simulink model "example_C_simulation_of_nominal_case"  (R2017b)
settings: Solver=VariableStepAuto  StartTime=0.0  StopTime=0.5  MaxStep=1e-3  RelTol=1e-3
undefined symbols (not defined in the file): DiscIntNeverNeededParam
settings Model: Creator=user  LastModifiedBy=user

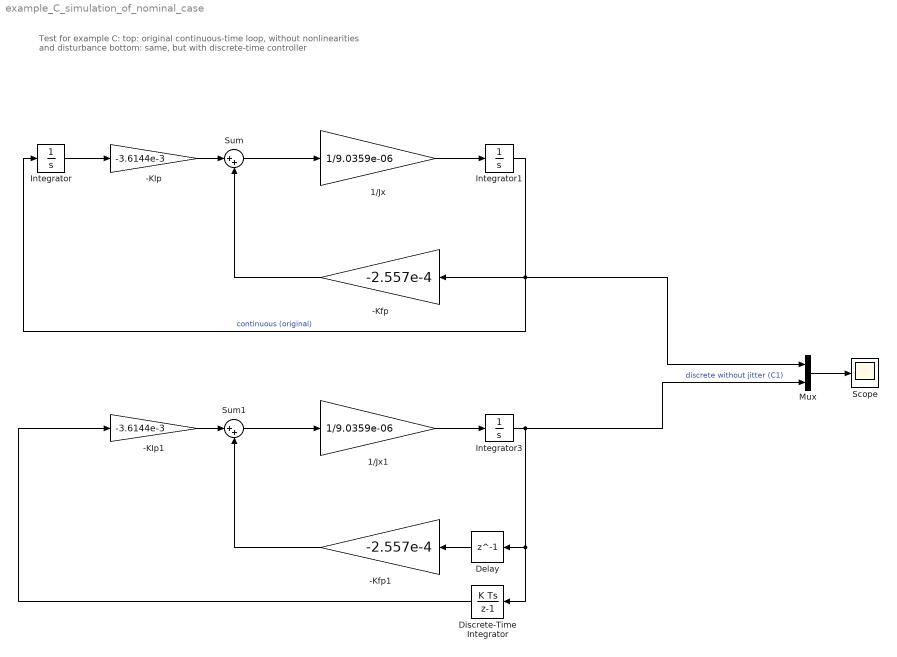
== system example_C_simulation_of_nominal_case ==
  note: Test for example C:
      | top: original continuous-time loop, without nonlinearities and disturbance
      | bottom: same, but with discrete-time controller
  -KIp : Gain  Gain=-3.6144e-3
  -KIp1 : Gain  Gain=-3.6144e-3
  -Kfp : Gain  Gain=-2.557e-4
  -Kfp1 : Gain  Gain=-2.557e-4
  1/Jx : Gain  Gain=1/9.0359e-06
  1/Jx1 : Gain  Gain=1/9.0359e-06
  Delay : Delay  DelayLength=1  SampleTime=0.01
  Discrete-Time Integrator : DiscreteIntegrator  gainval=1  InitialConditionSetting=State (most efficient)  SampleTime=0.01  ICPrevOutput=DiscIntNeverNeededParam  ICPrevScaledInput=DiscIntNeverNeededParam
  Integrator : Integrator
  Integrator1 : Integrator  InitialCondition=1
  Integrator3 : Integrator  InitialCondition=1
  Mux : Mux  Inputs=2
  Scope : Scope
  Sum : Sum  Inputs=|++
  Sum1 : Sum  Inputs=|++
  wires:
  Integrator/1 -> -KIp/1
  -KIp/1 -> Sum/1
  Sum/1 -> 1/Jx/1
  1/Jx/1 -> Integrator1/1
  Integrator1/1 -> -Kfp/1, Mux/1, Integrator/1  "continuous (original)"
  -Kfp/1 -> Sum/2
  -Kfp1/1 -> Sum1/2
  Integrator3/1 -> Mux/2, Delay/1, Discrete-Time Integrator/1  "discrete without jitter (C1)"
  1/Jx1/1 -> Integrator3/1
  Sum1/1 -> 1/Jx1/1
  -KIp1/1 -> Sum1/1
  Discrete-Time Integrator/1 -> -KIp1/1
  Delay/1 -> -Kfp1/1
  Mux/1 -> Scope/1
